simulink model "hummer_model_R2018a"  (R2018a)
settings: Solver=VariableStepAuto  StartTime=0.0  StopTime=10*60  RelTol=1e-3
libraries: simulink x1
settings Model: Creator=kjartan  LastModifiedBy=kjartan
settings DataIOCC: ReturnWorkspaceOutputs=on
settings SFSimCC: SimUseLocalCustomCode=on
settings RTWCC: RTWUseLocalCustomCode=on

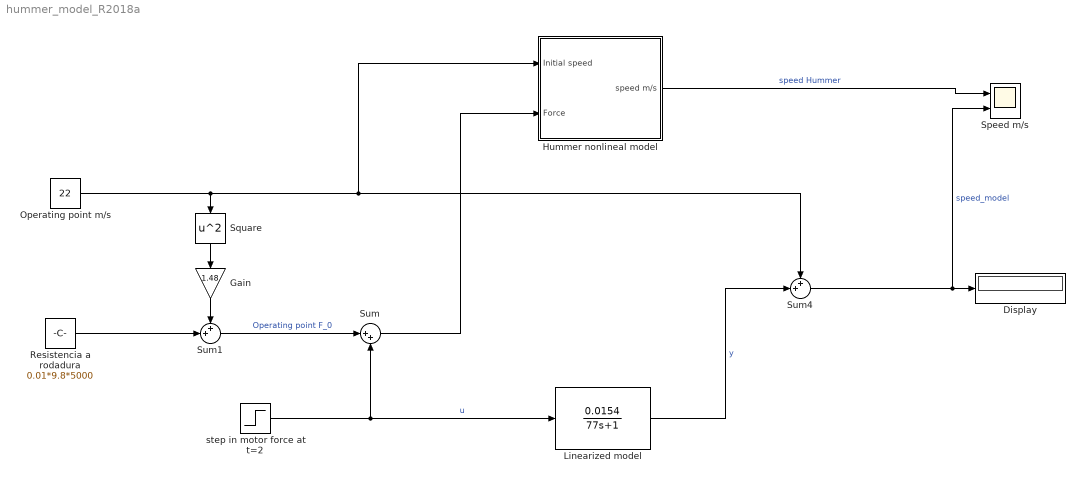
== system hummer_model_R2018a ==
  Display : Display
  Gain : Gain  Gain=1.48
  Hummer nonlineal model : Subsystem
  Linearized model : TransferFcn  Numerator=[0.0154]  Denominator=[77 1]
  Operating point m/s : Constant  Value=22
  Resistencia a rodadura : Constant  Value=0.01*9.8*5000
  Speed m/s : Scope  NumInputPorts=2
  Square : Math  Operator=square  SaturateOnIntegerOverflow=on
  Sum : Sum  Inputs=|++
  Sum1 : Sum  Inputs=++|
  Sum4 : Sum  Inputs=++|
  step in motor force at t=2 : Step  Time=2  After=100  SampleTime=0
  wires:
  Sum4/1 -> Speed m/s/2, Display/1  "speed_model"
  Hummer nonlineal model/1(speed m/s) -> Speed m/s/1  "speed Hummer"
  Linearized model/1 -> Sum4/2  "y"
  Operating point m/s/1 -> Square/1, Sum4/1, Hummer nonlineal model/1(Initial speed)
  Square/1 -> Gain/1
  Gain/1 -> Sum1/1
  Resistencia a rodadura/1 -> Sum1/2
  Sum1/1 -> Sum/1  "Operating point F_0"
  Sum/1 -> Hummer nonlineal model/2(Force)
  step in motor force at t=2/1 -> Sum/2, Linearized model/1  "u"

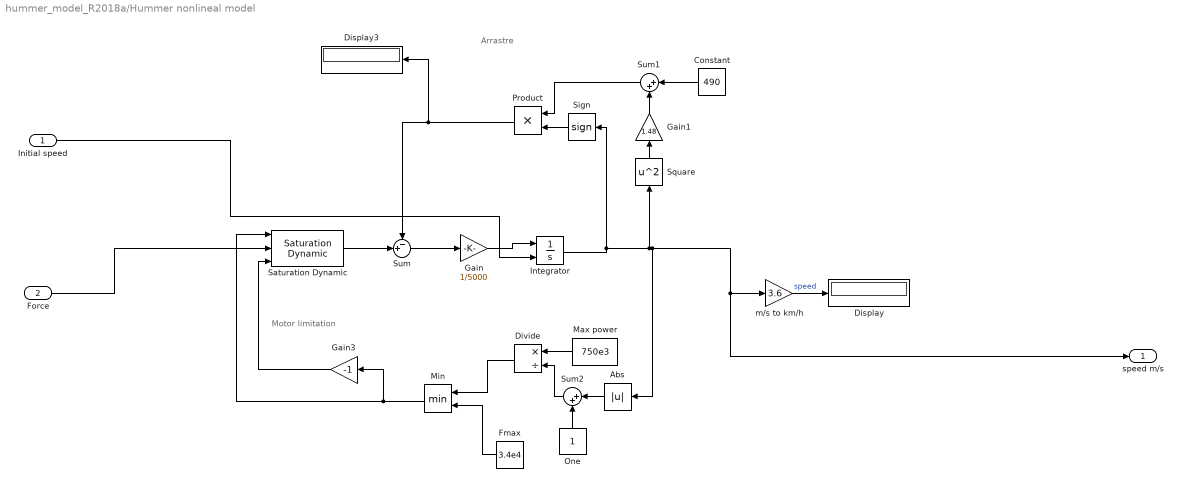
== system hummer_model_R2018a/Hummer nonlineal model ==
  note: Motor limitation
  note: Arrastre
  Initial speed : Inport
  Force : Inport  Port=2
  Abs : Abs
  Constant : Constant  Value=490
  Display : Display
  Display3 : Display
  Divide : Product  Inputs=*/
  Fmax : Constant  Value=3.4e4
  Gain : Gain  Gain=1/5000
  Gain1 : Gain  Gain=1.48
  Gain3 : Gain  Gain=-1
  Integrator : Integrator  InitialConditionSource=external
  Max power : Constant  Value=750e3
  Min : MinMax  Inputs=2
  One : Constant  OutDataTypeStr=Inherit: Inherit via back propagation
  Product : Product
  Saturation Dynamic : simulink/Discontinuities/Saturation Dynamic  OutMin=[]  OutMax=[]  OutDataTypeStr=Inherit: Same as second input  OutDataType=fixdt(1, 16)  OutScaling=2^-10  DoSatur=off
  Sign : Signum
  Square : Math  Operator=square  SaturateOnIntegerOverflow=on
  Sum : Sum  Inputs=-+|
  Sum1 : Sum  Inputs=|++
  Sum2 : Sum  Inputs=|++
  m/s to km/h : Gain  Gain=3.6
  speed m/s : Outport
  wires:
  Divide/1 -> Min/1
  Abs/1 -> Sum2/1
  Force/1 -> Saturation Dynamic/2
  m/s to km/h/1 -> Display/1  "speed"
  Square/1 -> Gain1/1
  Gain1/1 -> Sum1/2
  Sign/1 -> Product/2
  Constant/1 -> Sum1/1
  Sum/1 -> Gain/1
  Integrator/1 -> Abs/1, speed m/s/1, m/s to km/h/1, Square/1, Sign/1
  Sum1/1 -> Product/1
  Min/1 -> Gain3/1, Saturation Dynamic/1
  Initial speed/1 -> Integrator/2
  One/1 -> Sum2/2
  Fmax/1 -> Min/2
  Product/1 -> Sum/1, Display3/1
  Max power/1 -> Divide/1
  Gain/1 -> Integrator/1
  Gain3/1 -> Saturation Dynamic/3
  Saturation Dynamic/1 -> Sum/2
  Sum2/1 -> Divide/2
